simulink model "RTRCSystemValidation"  (R2022a)
settings: Solver=VariableStepAuto  StartTime=0.0  StopTime=TsimTime  FixedStep=Tsim  MaxStep=Tsim*100  RelTol=1e-5
undefined symbols (not defined in the file): Cdc, Fpwm, Jt, Kdw, Ke, Ki, Kii, Kiv, Kiw, Kp, Kpi, Kpv, Kpw, Krpm, Kt, Ktv, Ldc, Le, P, Rdc, Re, RPM_slope, Tload, Tpwm_buck, Vdc_c
libraries: simulink x10, slpidlib x1
settings Model: Creator=MasterGnome  LastModifiedBy=MasterGnome
settings SolverCC: ZeroCrossAlgorithm=Adaptive
settings DebuggingCC: IgnoredZcDiagnostic=none  UnconnectedInputMsg=warning  UnconnectedOutputMsg=warning  UnconnectedLineMsg=warning
settings RTWCC: DLArmComputeVersion=19.05

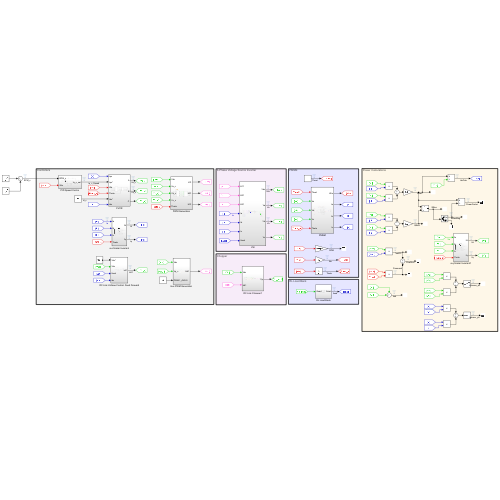
[thumbnail: Simulink's stored preview of the top-level diagram]
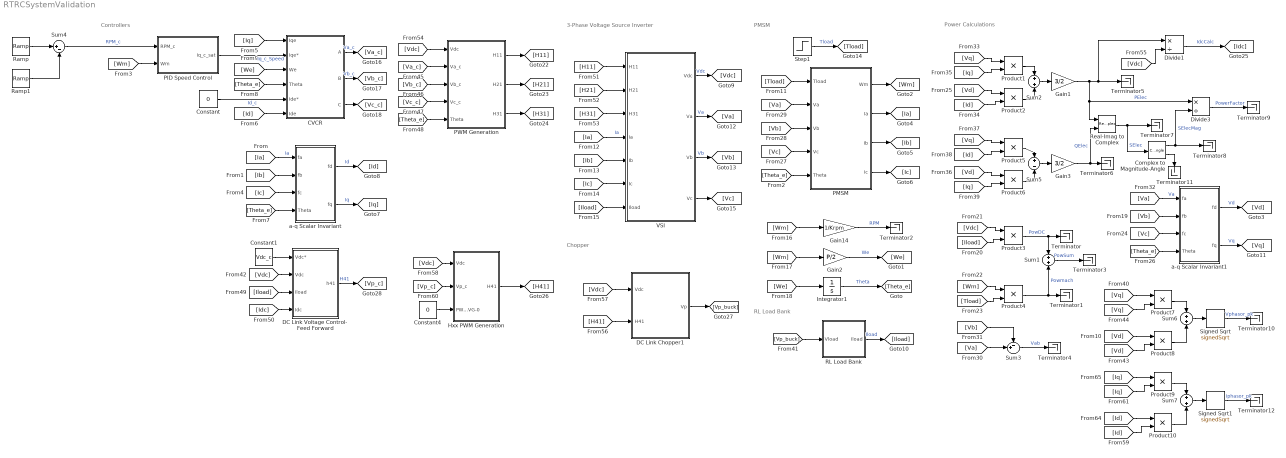
== system RTRCSystemValidation ==
  note: RL Load Bank
  note: Power Calculations
  note: PMSM
  note: Controllers
  note: 3-Phase Voltage Source Inverter
  note: Chopper
  CVCR : Subsystem
  Complex to Magnitude-Angle : ComplexToMagnitudeAngle
  Constant : Constant  Value=0
  Constant1 : Constant  Value=Vdc_c
  Constant4 : Constant  Value=0
  DC Link Chopper1 : Subsystem
  DC Link Voltage Control- Feed Forward : Subsystem
  Divide1 : Product  Inputs=*/
  Divide3 : Product  Inputs=*/
  Gain1 : Gain  Gain=3/2
  Gain14 : Gain  Gain=1/Krpm
  Gain2 : Gain  Gain=P/2
  Gain3 : Gain  Gain=3/2
  Hxx PWM Generation : Subsystem
  Integrator1 : Integrator
  PID Speed Control : Subsystem
  PMSM : Subsystem
  PWM Generation : Subsystem
  Product{1..10} (10 alike) : Product
  RL Load Bank : Subsystem
  Ramp : simulink/Sources/Ramp  slope=RPM_slope  start=RPM_Tstart  InitialOutput=0
  Ramp1 : simulink/Sources/Ramp  slope=RPM_slope  start=RPM_Tend  InitialOutput=0
  Real-Imag to Complex : RealImagToComplex
  Signed Sqrt : Sqrt  Operator=signedSqrt
  Signed Sqrt1 : Sqrt  Operator=signedSqrt
  Step1 : Step  Time=0.01  After=Tload  SampleTime=0
  Sum{1..2,6..7} (4 alike) : Sum  Inputs=+|+
  Sum3 : Sum  Inputs=-+|
  Sum4 : Sum  Inputs=|+-
  Sum5 : Sum  Inputs=+|-
  Terminator{,1..12} (13 alike) : Terminator
  VSI : Subsystem
  a-q Scalar Invariant : Subsystem
  a-q Scalar Invariant1 : Subsystem
  wires:
  Gain14/1 -> Terminator2/1  "RPM"
  PMSM/1(Wm) -> [Wm]
  Step1/1 -> [Tload]  "Tload"
  Gain2/1 -> [We]  "We"
  PMSM/2(Ia) -> [Ia]
  PMSM/3(Ib) -> [Ib]
  PMSM/4(Ic) -> [Ic]
  [Ia] -> a-q Scalar Invariant/1(fa)  "Ia"
  [Ib] -> a-q Scalar Invariant/2(fb)
  [Ic] -> a-q Scalar Invariant/3(fc)
  [Iq] -> CVCR/1(Iqe)
  [Id] -> CVCR/6(Ide)
  Integrator1/1 -> [Theta_e]  "Theta"
  [Theta_e] -> CVCR/4(Theta)
  [We] -> CVCR/3(We)
  Constant/1 -> CVCR/5(Ide*)  "Id_c"
  [Theta_e] -> PMSM/5(Theta)
  a-q Scalar Invariant/2(fq) -> [Iq]  "Iq"
  a-q Scalar Invariant/1(fd) -> [Id]  "Id"
  [Theta_e] -> a-q Scalar Invariant/4(Theta)
  Ramp/1 -> Sum4/1
  Ramp1/1 -> Sum4/2
  [Vdc] -> Product3/1
  [Iload] -> Product3/2
  Product3/1 -> Terminator/1, Sum1/1  "PowDC"
  Product4/1 -> Sum1/2, Terminator1/1  "Powmach"
  [Wm] -> Product4/1
  [Tload] -> Product4/2
  [Ib] -> VSI/5(Ib)
  [Ia] -> VSI/4(Ia)  "Ia"
  [Ic] -> VSI/6(Ic)
  VSI/1(Vdc) -> [Vdc]  "Vdc"
  [Tload] -> PMSM/1(Tload)
  Sum4/1 -> PID Speed Control/1(RPM_c)  "RPM_c"
  [Wm] -> PID Speed Control/2(Wm)
  PID Speed Control/1(Iq_c_sat) -> CVCR/2(Iqe*)  "Iq_c_Speed"
  [Wm] -> Gain14/1
  [Iload] -> VSI/7(Iload)
  [Wm] -> Gain2/1
  [We] -> Integrator1/1
  Sum1/1 -> Terminator3/1  "PowSum"
  Sum3/1 -> Terminator4/1  "Vab"
  [Vb] -> a-q Scalar Invariant1/2(fb)
  [Theta_e] -> a-q Scalar Invariant1/4(Theta)
  a-q Scalar Invariant1/1(fd) -> [Vd]  "Vd"
  [Vc] -> a-q Scalar Invariant1/3(fc)
  a-q Scalar Invariant1/2(fq) -> [Vq]  "Vq"
  [Va] -> a-q Scalar Invariant1/1(fa)  "Va"
  VSI/2(Va) -> [Va]  "Va"
  VSI/3(Vb) -> [Vb]  "Vb"
  VSI/4(Vc) -> [Vc]
  [Vc] -> PMSM/4(Vc)
  [Vb] -> PMSM/3(Vb)
  [Va] -> PMSM/2(Va)
  [Va] -> Sum3/2
  [Vb] -> Sum3/1
  [Iq] -> Product1/2
  [Vq] -> Product1/1
  [Id] -> Product2/2
  [Vd] -> Product2/1
  Product1/1 -> Sum2/1
  Product2/1 -> Sum2/2
  Sum2/1 -> Gain1/1
  Gain1/1 -> Divide1/1, Terminator5/1, Real-Imag to Complex/1, Divide3/1  "PElec"
  Product6/1 -> Sum5/2
  Product5/1 -> Sum5/1
  Gain3/1 -> Real-Imag to Complex/2, Terminator6/1  "QElec"
  [Vd] -> Product6/1
  [Vq] -> Product5/1
  Sum5/1 -> Gain3/1
  [Iq] -> Product6/2
  [Id] -> Product5/2
  Real-Imag to Complex/1 -> Complex to Magnitude-Angle/1, Terminator7/1  "SElec"
  Complex to Magnitude-Angle/1 -> Divide3/2, Terminator8/1  "SElecMag"
  Divide3/1 -> Terminator9/1  "PowerFactor"
  CVCR/3(C) -> [Vc_c]
  CVCR/2(B) -> [Vb_c]  "Vb_c"
  CVCR/1(A) -> [Va_c]  "Va_c"
  [H21] -> VSI/2(H21)
  [H31] -> VSI/3(H31)
  RL Load Bank/1(Iload) -> [Iload]  "Iload"
  [H11] -> VSI/1(H11)
  Complex to Magnitude-Angle/2 -> Terminator11/1
  [Vdc] -> PWM Generation/1(Vdc)
  [Va_c] -> PWM Generation/2(Va_c)
  [Vb_c] -> PWM Generation/3(Vb_c)
  [Vc_c] -> PWM Generation/4(Vc_c)
  [Theta_e] -> PWM Generation/5(Theta)
  PWM Generation/1(H11) -> [H11]
  PWM Generation/2(H21) -> [H21]
  PWM Generation/3(H31) -> [H31]
  [Vp_buck] -> RL Load Bank/1(Vload)
  Constant1/1 -> DC Link Voltage Control- Feed Forward/1(Vdc*)
  [Vdc] -> DC Link Voltage Control- Feed Forward/2(Vdc)
  [Iload] -> DC Link Voltage Control- Feed Forward/3(Iload)
  DC Link Voltage Control- Feed Forward/1(h41) -> [Vp_c]  "H41"
  [Vdc] -> Divide1/2
  [Idc] -> DC Link Voltage Control- Feed Forward/4(Idc)
  Divide1/1 -> [Idc]  "IdcCalc"
  Hxx PWM Generation/1(H41) -> [H41]
  Constant4/1 -> Hxx PWM Generation/3(PWM-1_AVG-0)
  [Vp_c] -> Hxx PWM Generation/2(Vp_c)
  [Vdc] -> Hxx PWM Generation/1(Vdc)
  [Vdc] -> DC Link Chopper1/1(Vdc)
  [H41] -> DC Link Chopper1/2(H41)
  DC Link Chopper1/1(Vp) -> [Vp_buck]
  [Vq] -> Product7/1
  [Vd] -> Product8/1
  Product7/1 -> Sum6/1
  Product8/1 -> Sum6/2
  [Vd] -> Product8/2
  [Vq] -> Product7/2
  Sum6/1 -> Signed Sqrt/1
  Signed Sqrt/1 -> Terminator10/1  "Vphasor_pk"
  Product9/1 -> Sum7/1
  Product10/1 -> Sum7/2
  Sum7/1 -> Signed Sqrt1/1
  Signed Sqrt1/1 -> Terminator12/1  "Iphasor_pk"
  [Iq] -> Product9/1
  [Id] -> Product10/1
  [Id] -> Product10/2
  [Iq] -> Product9/2

== system RTRCSystemValidation/CVCR ==
  Iqe : Inport
  Iqe* : Inport  Port=2
  We : Inport  Port=3
  Theta : Inport  Port=4
  Ide* : Inport  Port=5
  Ide : Inport  Port=6
  "CVCR " : Subsystem
  q-a Scalar Invariant : Subsystem
  A : Outport
  B : Outport  Port=2
  C : Outport  Port=3
  wires:
  q-a Scalar Invariant/3(c) -> C/1
  We/1 -> "CVCR "/3(We)
  Theta/1 -> q-a Scalar Invariant/3(theta)
  q-a Scalar Invariant/1(a) -> A/1
  q-a Scalar Invariant/2(b) -> B/1
  Iqe/1 -> "CVCR "/1(Iq)
  Iqe*/1 -> "CVCR "/2(Iq_c)
  Ide*/1 -> "CVCR "/4(Id_c)
  Ide/1 -> "CVCR "/5(Id)
  "CVCR "/1(Vqe) -> q-a Scalar Invariant/1(fq)  "Vq*"
  "CVCR "/2(Vde) -> q-a Scalar Invariant/2(fd)  "Vd*"

== system RTRCSystemValidation/DC Link Chopper1 ==
  Vdc : Inport
  H41 : Inport  Port=2
  Divide : Product  Inputs=**
  Vp : Outport
  wires:
  H41/1 -> [H41]
  [Vp] -> Vp/1
  Vdc/1 -> [Vdc]
  [H41] -> Divide/2
  [Vdc] -> Divide/1
  Divide/1 -> [Vp]  "Vp"

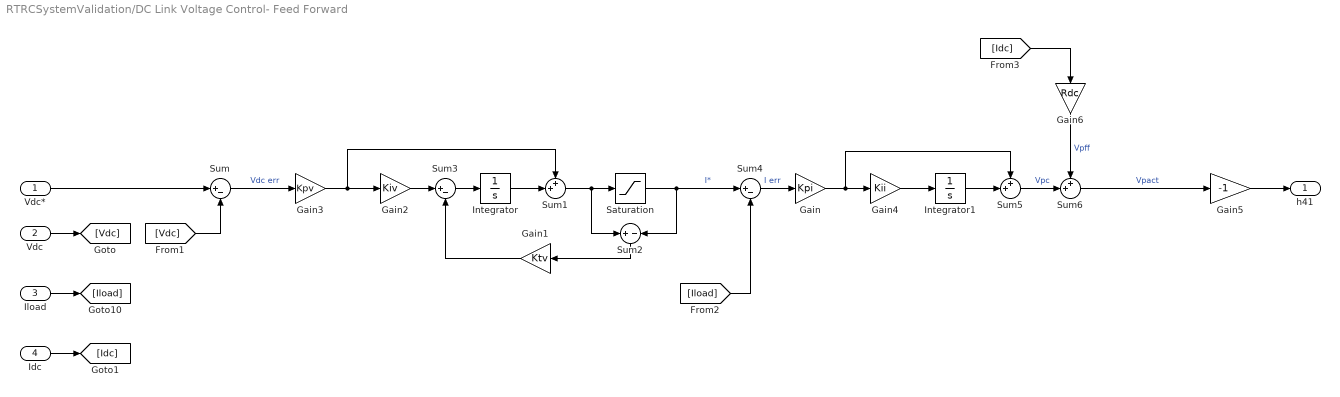
== system RTRCSystemValidation/DC Link Voltage Control- Feed Forward ==
  Vdc* : Inport
  Vdc : Inport  Port=2
  Iload : Inport  Port=3
  Idc : Inport  Port=4
  Gain : Gain  Gain=Kpi
  Gain1 : Gain  Gain=Ktv
  Gain2 : Gain  Gain=Kiv
  Gain3 : Gain  Gain=Kpv
  Gain4 : Gain  Gain=Kii
  Gain5 : Gain  Gain=-1
  Gain6 : Gain  Gain=Rdc
  Integrator : Integrator
  Integrator1 : Integrator
  Saturation : Saturate  UpperLimit=0  LowerLimit=-200
  Sum : Sum  Inputs=|+-
  Sum1 : Sum  Inputs=++|
  Sum2 : Sum  Inputs=+|-
  Sum3 : Sum  Inputs=|+-
  Sum4 : Sum  Inputs=|+-
  Sum5 : Sum  Inputs=++|
  Sum6 : Sum  Inputs=++|
  h41 : Outport
  wires:
  Sum/1 -> Gain3/1  "Vdc err"
  Gain3/1 -> Gain2/1, Sum1/1
  Sum1/1 -> Saturation/1, Sum2/1
  Gain2/1 -> Sum3/1
  Integrator/1 -> Sum1/2
  Sum3/1 -> Integrator/1
  Gain1/1 -> Sum3/2
  Sum2/1 -> Gain1/1
  Vdc*/1 -> Sum/1
  Sum4/1 -> Gain/1  "I err"
  Vdc/1 -> [Vdc]
  [Vdc] -> Sum/2
  Iload/1 -> [Iload]
  [Iload] -> Sum4/2
  Gain/1 -> Gain4/1, Sum5/1
  Gain4/1 -> Integrator1/1
  Integrator1/1 -> Sum5/2
  Gain5/1 -> h41/1
  Sum5/1 -> Sum6/2  "Vpc"
  Saturation/1 -> Sum4/1, Sum2/2  "I*"
  Idc/1 -> [Idc]
  Sum6/1 -> Gain5/1  "Vpact"
  [Idc] -> Gain6/1
  Gain6/1 -> Sum6/1  "Vpff"

== system RTRCSystemValidation/Hxx PWM Generation ==
  Vdc : Inport
  Vp_c : Inport  Port=2
  PWM-1_AVG-0 : Inport  Port=3
  Avg Model : Subsystem
  Switch7 : Switch  Criteria=u2 > Threshold  ZeroCross=off  SaturateOnIntegerOverflow=off  InputSameDT=off
  Switching Model : Subsystem
  H41 : Outport
  wires:
  [Vdc] -> Avg Model/1(Vdc)
  [Vp_c] -> Avg Model/2(Vp_c)
  Avg Model/1(H41_avg) -> [H41_avg]
  [Vdc] -> Switching Model/1(Vdc)
  [Vp_c] -> Switching Model/2(Vp_c)
  Switching Model/1(H41_pwm) -> [H41_pwm]
  [PWM_AVG] -> Switch7/2
  Switch7/1 -> [H41]
  [H41_pwm] -> Switch7/1
  [H41_avg] -> Switch7/3
  Vp_c/1 -> [Vp_c]
  Vdc/1 -> [Vdc]
  [H41] -> H41/1
  PWM-1_AVG-0/1 -> [PWM_AVG]

== system RTRCSystemValidation/PID Speed Control ==
  RPM_c : Inport
  Wm : Inport  Port=2
  Derivative : Derivative
  Gain1 : Gain  Gain=Kdw
  Gain10 : Gain  Gain=Kpw
  Gain11 : Gain  Gain=Krpm
  Gain2 : Gain  Gain=Kiw
  Integrator2 : Integrator
  Kt : Gain  Gain=100
  PID Controller : slpidlib/PID Controller  Controller=PID  Form=Parallel  TimeDomain=Continuous-time  UseExternalTs=off  SampleTime=-1  IntegratorMethod=Forward Euler  FilterMethod=Forward Euler  ControllerParametersSource=internal  P=Kpw  I=Kiw  UseKiTs=off  D=Kdw  N=100  UseFilter=on  TunerSelectOption=Transfer Function Based (PID Tuner App)  InitialConditionSource=internal  InitialConditionForIntegrator=0  InitialConditionForFilter=0  DifferentiatorICPrevScaledInput=0  ExternalReset=none  TrackingMode=off  Kt=1  LimitOutput=off  SatLimitsSource=internal  UpperSaturationLimit=inf  LowerSaturationLimit=-inf  LinearizeAsGain=on  AntiWindupMode=none  Kb=1  POutMin=[]  POutMax=[]  IOutMin=[]  IOutMax=[]  DOutMin=[]  DOutMax=[]  NOutMin=[]  NOutMax=[]  SumOutMin=[]  SumOutMax=[]  SaturationOutMin=[]  SaturationOutMax=[]  PParamMin=[]  PParamMax=[]  IParamMin=[]  IParamMax=[]  DParamMin=[]  DParamMax=[]  NParamMin=[]  NParamMax=[]  KbParamMin=[]  KbParamMax=[]  KtParamMin=[]  KtParamMax=[]  KbOutMin=[]  KbOutMax=[]  KtOutMin=[]  KtOutMax=[]  IntegratorOutMin=[]  IntegratorOutMax=[]  FilterOutMin=[]  FilterOutMax=[]  SumI1OutMin=[]  SumI1OutMax=[]  SumI2OutMin=[]  SumI2OutMax=[]  SumI3OutMin=[]  SumI3OutMax=[]  SumI4OutMin=[]  SumI4OutMax=[]  SumDOutMin=[]  SumDOutMax=[]  DifferentiatorOutMin=[]  DifferentiatorOutMax=[]  FilterDiffOutCoefMin=[]  FilterDiffOutCoefMax=[]  ReciprocalOutMin=[]  ReciprocalOutMax=[]  SumDenOutMin=[]  SumDenOutMax=[]  SumNumOutMin=[]  SumNumOutMax=[]  DivideOutMin=[]  DivideOutMax=[]  UdiffTsProdOutMin=[]  UdiffTsProdOutMax=[]  NTsProdOutMin=[]  NTsProdOutMax=[]  UintegralTsProdOutMin=[]  UintegralTsProdOutMax=[]  UngainTsProdOutMin=[]  UngainTsProdOutMax=[]  IntegratorContinuousStateAttributes=''  IntegratorStateMustResolveToSignalObject=off  IntegratorRTWStateStorageClass=Auto  FilterContinuousStateAttributes=''  FilterStateMustResolveToSignalObject=off  FilterRTWStateStorageClass=Auto  ParallelPVariant=InternalParameters  IdealPVariant=Disabled  IVariant=InternalParameters  DVariant=InternalParameters  IntegratorVariant=Continuous  SatVariant=Disabled  AWVariant=Passthrough  PCopyVariant=Disabled  TRVariant=Disabled  FdbkBlocksVariant=Forward  IdealPFdbkVariant=Disabled  SatFdbkVariant=Disabled  DerivativeFilterVariant=ContFilter  NVariant=InternalParameters  NCopyVariant=Disabled  FilterICVariant=InternalICsFilter  IntegratorICVariant=InternalICs  ExternalResetVariant=Disabled  TRSumVariant=Passthrough  SumFdbkVariant=Disabled  SumVariant=Sum_PID  TsampFilterVariant=InternalTs  TsampNgainVariant=Passthrough  TsampIntegralVariant=Passthrough  ExternalSaturationOutDataTypeStr=Inherit: Same as second input  aMode=0
  Saturation : Saturate  UpperLimit=150  LowerLimit=-150
  Saturation1 : Saturate  UpperLimit=150  LowerLimit=-150
  Sum1 : Sum  Inputs=+++
  Sum2 : Sum  Inputs=++|
  Sum3 : Sum  Inputs=|+-
  Sum4 : Sum  Inputs=+|-
  Sum5 : Sum  Inputs=|+-
  Sum9 : Sum  Inputs=|+-
  Iq_c_sat : Outport
  wires:
  Gain10/1 -> Sum1/1
  Wm/1 -> Sum9/2
  Gain1/1 -> Sum3/1
  Derivative/1 -> Sum1/2
  Gain11/1 -> Sum9/1
  RPM_c/1 -> Gain11/1
  Sum3/1 -> Derivative/1
  Sum5/1 -> Integrator2/1
  Saturation1/1 -> Sum1/3, Sum4/2
  Sum4/1 -> Kt/1
  Kt/1 -> Sum5/2
  Gain2/1 -> Sum5/1
  Integrator2/1 -> Sum2/2
  Sum9/1 -> PID Controller/1, Gain2/1, Gain1/1, Gain10/1
  Sum2/1 -> Sum4/1, Saturation1/1  "Iq_c"
  PID Controller/1 -> Saturation/1
  Saturation/1 -> Iq_c_sat/1  "Iq_c_sat"
  Sum1/1 -> ?  "Iq_c"

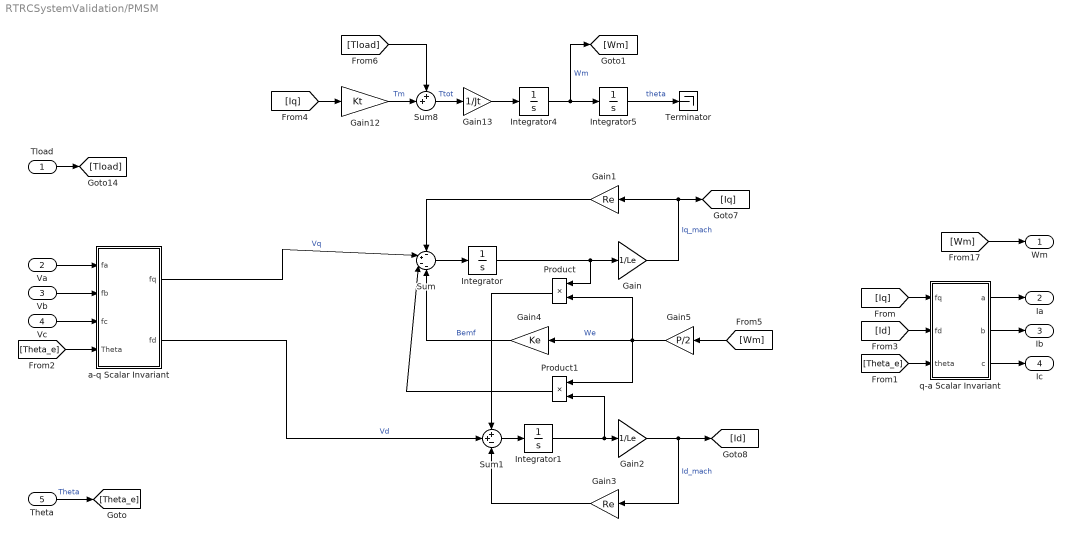
== system RTRCSystemValidation/PMSM ==
  Tload : Inport
  Va : Inport  Port=2
  Vb : Inport  Port=3
  Vc : Inport  Port=4
  Theta : Inport  Port=5
  Gain : Gain  Gain=1/Le
  Gain1 : Gain  Gain=Re
  Gain12 : Gain  Gain=Kt
  Gain13 : Gain  Gain=1/Jt
  Gain2 : Gain  Gain=1/Le
  Gain3 : Gain  Gain=Re
  Gain4 : Gain  Gain=Ke
  Gain5 : Gain  Gain=P/2
  Integrator{,1,4..5} (4 alike) : Integrator
  Product : Product
  Product1 : Product
  Sum : Sum  Inputs=-+--
  Sum1 : Sum  Inputs=++-
  Sum8 : Sum  Inputs=++|
  Terminator : Terminator
  a-q Scalar Invariant : Subsystem
  q-a Scalar Invariant : Subsystem
  Wm : Outport
  Ia : Outport  Port=2
  Ib : Outport  Port=3
  Ic : Outport  Port=4
  wires:
  Sum1/1 -> Integrator1/1
  Gain5/1 -> Product1/1, Product/2, Gain4/1  "We"
  Gain1/1 -> Sum/1
  Integrator4/1 -> [Wm], Integrator5/1  "Wm"
  Sum8/1 -> Gain13/1  "Ttot"
  Integrator1/1 -> Product1/2, Gain2/1
  Gain3/1 -> Sum1/3
  [Tload] -> Sum8/1
  Integrator/1 -> Product/1, Gain/1
  Gain13/1 -> Integrator4/1
  Gain4/1 -> Sum/4  "Bemf"
  Sum/1 -> Integrator/1
  Product/1 -> Sum1/1
  Integrator5/1 -> Terminator/1  "theta"
  Product1/1 -> Sum/3
  a-q Scalar Invariant/1(fq) -> Sum/2  "Vq"
  q-a Scalar Invariant/3(c) -> Ic/1
  q-a Scalar Invariant/1(a) -> Ia/1
  Gain2/1 -> [Id], Gain3/1  "Id_mach"
  q-a Scalar Invariant/2(b) -> Ib/1
  Gain/1 -> [Iq], Gain1/1  "Iq_mach"
  Vc/1 -> a-q Scalar Invariant/3(fc)
  Vb/1 -> a-q Scalar Invariant/2(fb)
  Va/1 -> a-q Scalar Invariant/1(fa)
  a-q Scalar Invariant/2(fd) -> Sum1/2  "Vd"
  [Theta_e] -> a-q Scalar Invariant/4(Theta)
  [Theta_e] -> q-a Scalar Invariant/3(theta)
  Theta/1 -> [Theta_e]  "Theta"
  [Iq] -> q-a Scalar Invariant/1(fq)
  [Id] -> q-a Scalar Invariant/2(fd)
  [Iq] -> Gain12/1
  Gain12/1 -> Sum8/2  "Tm"
  [Wm] -> Wm/1
  [Wm] -> Gain5/1
  Tload/1 -> [Tload]

== system RTRCSystemValidation/PWM Generation ==
  Vdc : Inport
  Va_c : Inport  Port=2
  Vb_c : Inport  Port=3
  Vc_c : Inport  Port=4
  Theta : Inport  Port=5
  "1-PWM, 0-AVG" : Constant  Value=0
  Hxx Avg PWM : Subsystem
  Modulation : Subsystem
  H11 : Outport
  H21 : Outport  Port=2
  H31 : Outport  Port=3
  wires:
  Modulation/1(Va_mod) -> [Va_mod]
  Modulation/2(Vb_mod) -> [Vb_mod]
  Hxx Avg PWM/1(H11) -> H11/1
  [Vb_mod] -> Hxx Avg PWM/3(Vb_mod)
  Hxx Avg PWM/2(H21) -> H21/1
  [Vc_mod] -> Hxx Avg PWM/4(Vc_mod)
  Modulation/3(Vc_mod) -> [Vc_mod]
  [Va_mod] -> Hxx Avg PWM/2(Va_mod)
  [Vdc] -> Hxx Avg PWM/1(Vdc)
  "1-PWM, 0-AVG"/1 -> Hxx Avg PWM/5(PWM-1_AVG-0)
  Hxx Avg PWM/3(H31) -> H31/1
  Vdc/1 -> [Vdc], Modulation/1(Vdc)
  Va_c/1 -> Modulation/2(Va_c)
  Vb_c/1 -> Modulation/3(Vb_c)
  Theta/1 -> Modulation/5(Theta)
  Vc_c/1 -> Modulation/4(Vc_c)

== system RTRCSystemValidation/RL Load Bank ==
  Vload : Inport
  Gain1 : Gain  Gain=-1
  Gain4 : Gain  Gain=1/Ldc
  Gain5 : Gain  Gain=Rdc
  Integrator2 : Integrator
  Sum6 : Sum  Inputs=|+-
  Iload : Outport
  wires:
  Gain5/1 -> Sum6/2
  Sum6/1 -> Gain4/1
  Vload/1 -> Sum6/1
  Gain4/1 -> Integrator2/1
  Integrator2/1 -> Gain1/1, Gain5/1  "Iload"
  Gain1/1 -> Iload/1

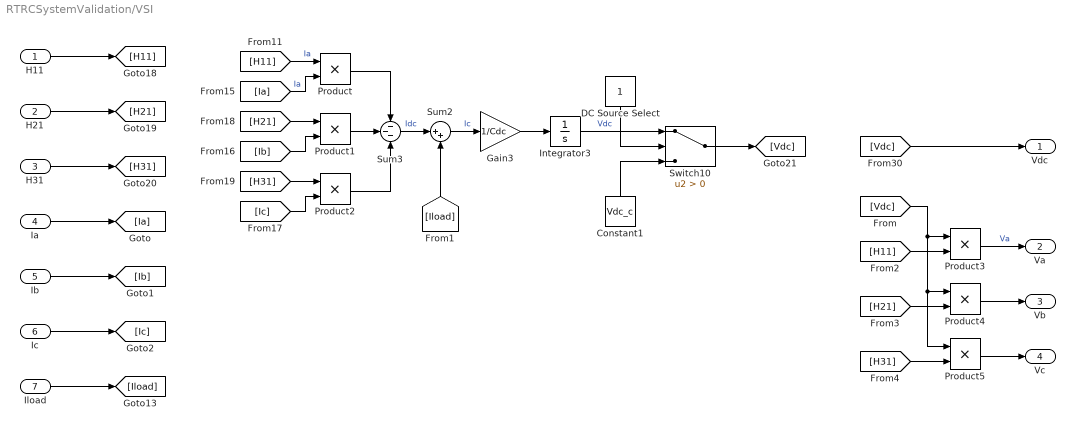
== system RTRCSystemValidation/VSI ==
  H11 : Inport
  H21 : Inport  Port=2
  H31 : Inport  Port=3
  Ia : Inport  Port=4
  Ib : Inport  Port=5
  Ic : Inport  Port=6
  Iload : Inport  Port=7
  Constant1 : Constant  Value=Vdc_c
  DC Source Select : Constant
  Gain3 : Gain  Gain=1/Cdc
  Integrator3 : Integrator  InitialCondition=Vdc_c/2
  Product{,1..5} (6 alike) : Product
  Sum2 : Sum  Inputs=|++
  Sum3 : Sum  Inputs=---
  Switch10 : Switch  Criteria=u2 > Threshold  ZeroCross=off  SaturateOnIntegerOverflow=off  InputSameDT=off
  Vdc : Outport
  Va : Outport  Port=2
  Vb : Outport  Port=3
  Vc : Outport  Port=4
  wires:
  Iload/1 -> [Iload]
  Sum3/1 -> Sum2/1  "Idc"
  H31/1 -> [H31]
  Sum2/1 -> Gain3/1  "Ic"
  H21/1 -> [H21]
  Product3/1 -> Va/1  "Va"
  [Ia] -> Product/2  "Ia"
  Product1/1 -> Sum3/2
  [Ib] -> Product1/2
  [H31] -> Product2/1
  [Ic] -> Product2/2
  Product2/1 -> Sum3/3
  [H21] -> Product1/1
  [Vdc] -> Vdc/1
  H11/1 -> [H11]
  [Vdc] -> Product3/1, Product5/1, Product4/1
  Product/1 -> Sum3/1
  [H11] -> Product/1  "Ia"
  Gain3/1 -> Integrator3/1
  Ib/1 -> [Ib]
  Ia/1 -> [Ia]
  Ic/1 -> [Ic]
  [Iload] -> Sum2/2
  Product4/1 -> Vb/1
  Product5/1 -> Vc/1
  Switch10/1 -> [Vdc]
  DC Source Select/1 -> Switch10/2
  Integrator3/1 -> Switch10/1  "Vdc"
  Constant1/1 -> Switch10/3
  [H11] -> Product3/2
  [H21] -> Product4/2
  [H31] -> Product5/2

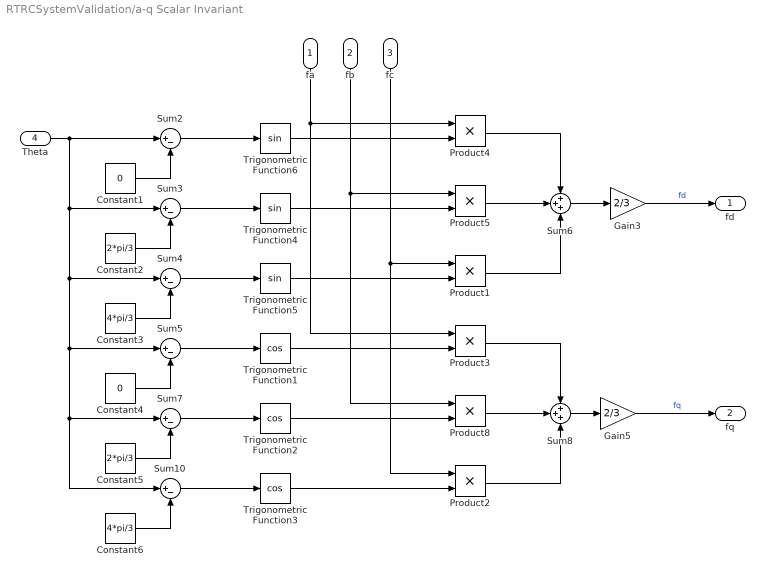
== system RTRCSystemValidation/a-q Scalar Invariant ==
  fa : Inport
  fb : Inport  Port=2
  fc : Inport  Port=3
  Theta : Inport  Port=4
  Constant1 : Constant  Value=0
  Constant2 : Constant  Value=2*pi/3
  Constant3 : Constant  Value=4*pi/3
  Constant4 : Constant  Value=0
  Constant5 : Constant  Value=2*pi/3
  Constant6 : Constant  Value=4*pi/3
  Gain3 : Gain  Gain=2/3
  Gain5 : Gain  Gain=2/3
  Product{1..5,8} (6 alike) : Product
  Sum{2..5,7,10} (6 alike) : Sum  Inputs=|+-
  Sum6 : Sum  Inputs=+++
  Sum8 : Sum  Inputs=+++
  Trigonometric Function1 : Trigonometry  Operator=cos
  Trigonometric Function2 : Trigonometry  Operator=cos
  Trigonometric Function3 : Trigonometry  Operator=cos
  Trigonometric Function4 : Trigonometry
  Trigonometric Function5 : Trigonometry
  Trigonometric Function6 : Trigonometry
  fd : Outport
  fq : Outport  Port=2
  wires:
  Product1/1 -> Sum6/3
  fc/1 -> Product2/1, Product1/1
  Sum4/1 -> Trigonometric Function5/1
  Constant5/1 -> Sum7/2
  Trigonometric Function4/1 -> Product5/2
  Sum7/1 -> Trigonometric Function2/1
  Constant6/1 -> Sum10/2
  Trigonometric Function3/1 -> Product2/2
  Theta/1 -> Sum10/1, Sum7/1, Sum5/1, Sum4/1, Sum3/1, Sum2/1
  Sum10/1 -> Trigonometric Function3/1
  Sum5/1 -> Trigonometric Function1/1
  Product2/1 -> Sum8/3
  Trigonometric Function2/1 -> Product8/2
  Product3/1 -> Sum8/1
  Constant3/1 -> Sum4/2
  Trigonometric Function6/1 -> Product4/2
  Product8/1 -> Sum8/2
  Trigonometric Function5/1 -> Product1/2
  Constant2/1 -> Sum3/2
  Sum3/1 -> Trigonometric Function4/1
  Sum8/1 -> Gain5/1
  Constant4/1 -> Sum5/2
  Constant1/1 -> Sum2/2
  Sum2/1 -> Trigonometric Function6/1
  fa/1 -> Product4/1, Product3/1
  Gain3/1 -> fd/1  "fd"
  Sum6/1 -> Gain3/1
  Trigonometric Function1/1 -> Product3/2
  Product4/1 -> Sum6/1
  Gain5/1 -> fq/1  "fq"
  fb/1 -> Product5/1, Product8/1
  Product5/1 -> Sum6/2

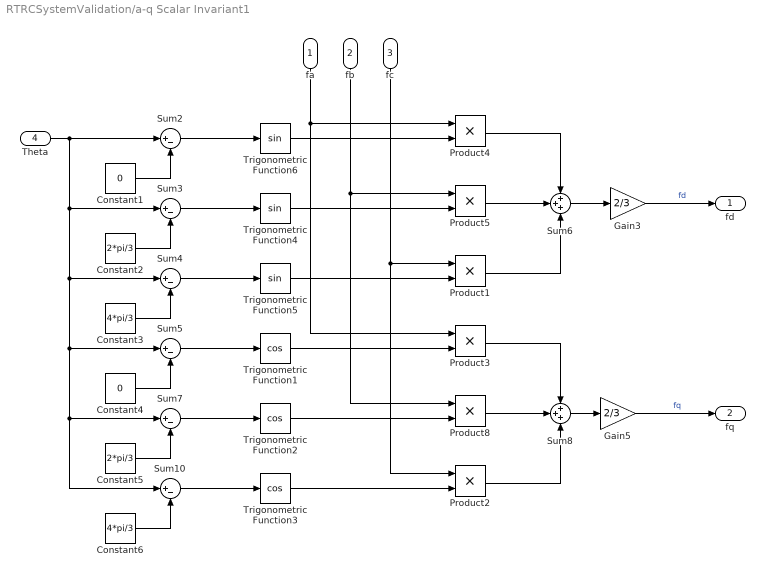
== system RTRCSystemValidation/a-q Scalar Invariant1 ==
  fa : Inport
  fb : Inport  Port=2
  fc : Inport  Port=3
  Theta : Inport  Port=4
  Constant1 : Constant  Value=0
  Constant2 : Constant  Value=2*pi/3
  Constant3 : Constant  Value=4*pi/3
  Constant4 : Constant  Value=0
  Constant5 : Constant  Value=2*pi/3
  Constant6 : Constant  Value=4*pi/3
  Gain3 : Gain  Gain=2/3
  Gain5 : Gain  Gain=2/3
  Product{1..5,8} (6 alike) : Product
  Sum{2..5,7,10} (6 alike) : Sum  Inputs=|+-
  Sum6 : Sum  Inputs=+++
  Sum8 : Sum  Inputs=+++
  Trigonometric Function1 : Trigonometry  Operator=cos
  Trigonometric Function2 : Trigonometry  Operator=cos
  Trigonometric Function3 : Trigonometry  Operator=cos
  Trigonometric Function4 : Trigonometry
  Trigonometric Function5 : Trigonometry
  Trigonometric Function6 : Trigonometry
  fd : Outport
  fq : Outport  Port=2
  wires:
  Product1/1 -> Sum6/3
  fc/1 -> Product2/1, Product1/1
  Sum4/1 -> Trigonometric Function5/1
  Constant5/1 -> Sum7/2
  Trigonometric Function4/1 -> Product5/2
  Sum7/1 -> Trigonometric Function2/1
  Constant6/1 -> Sum10/2
  Trigonometric Function3/1 -> Product2/2
  Theta/1 -> Sum10/1, Sum7/1, Sum5/1, Sum4/1, Sum3/1, Sum2/1
  Sum10/1 -> Trigonometric Function3/1
  Sum5/1 -> Trigonometric Function1/1
  Product2/1 -> Sum8/3
  Trigonometric Function2/1 -> Product8/2
  Product3/1 -> Sum8/1
  Constant3/1 -> Sum4/2
  Trigonometric Function6/1 -> Product4/2
  Product8/1 -> Sum8/2
  Trigonometric Function5/1 -> Product1/2
  Constant2/1 -> Sum3/2
  Sum3/1 -> Trigonometric Function4/1
  Sum8/1 -> Gain5/1
  Constant4/1 -> Sum5/2
  Constant1/1 -> Sum2/2
  Sum2/1 -> Trigonometric Function6/1
  fa/1 -> Product4/1, Product3/1
  Gain3/1 -> fd/1  "fd"
  Sum6/1 -> Gain3/1
  Trigonometric Function1/1 -> Product3/2
  Product4/1 -> Sum6/1
  Gain5/1 -> fq/1  "fq"
  fb/1 -> Product5/1, Product8/1
  Product5/1 -> Sum6/2

== system RTRCSystemValidation/CVCR/CVCR  ==
  Iq : Inport
  Iq_c : Inport  Port=2
  We : Inport  Port=3
  Id_c : Inport  Port=4
  Id : Inport  Port=5
  Gain6 : Gain  Gain=Ki
  Gain7 : Gain  Gain=Kp
  Gain8 : Gain  Gain=Ki
  Gain9 : Gain  Gain=Kp
  Integrator2 : Integrator
  Integrator3 : Integrator
  Product2 : Product
  Product3 : Product
  Sum2 : Sum  Inputs=++|
  Sum3 : Sum  Inputs=|++
  Sum4 : Sum  Inputs=-+|
  Sum5 : Sum  Inputs=|+-
  Sum6 : Sum  Inputs=|++
  Sum7 : Sum  Inputs=-+|
  Vqe : Outport
  Vde : Outport  Port=2
  wires:
  We/1 -> Product2/2, Product3/1
  Gain9/1 -> Product2/1, Gain8/1, Sum3/2
  Sum5/1 -> Gain9/1
  Integrator3/1 -> Sum3/1
  Product2/1 -> Sum6/2
  Gain7/1 -> Gain6/1, Sum2/1, Product3/2
  Product3/1 -> Sum7/1
  Sum6/1 -> Integrator2/1
  Id/1 -> Sum5/2
  Iq_c/1 -> Sum4/2
  Integrator2/1 -> Sum2/2
  Gain8/1 -> Sum7/2
  Sum4/1 -> Gain7/1
  Sum7/1 -> Integrator3/1
  Gain6/1 -> Sum6/1
  Iq/1 -> Sum4/1
  Sum2/1 -> Vqe/1  "Vqe"
  Id_c/1 -> Sum5/1
  Sum3/1 -> Vde/1  "Vde"

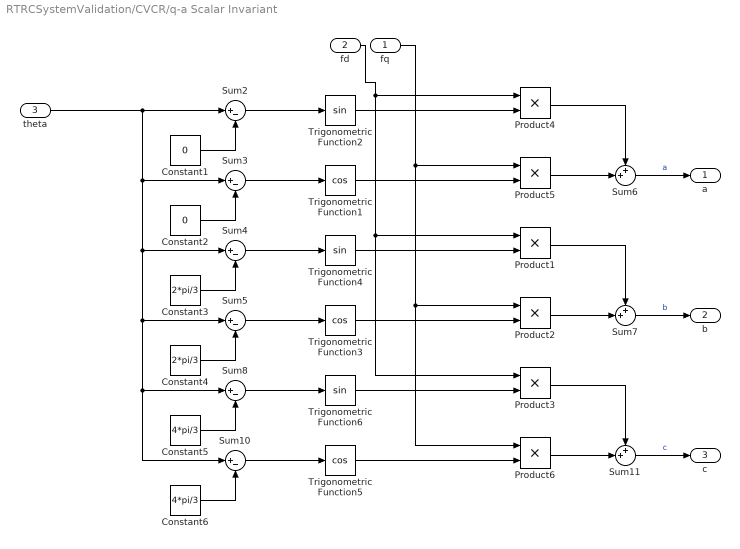
== system RTRCSystemValidation/CVCR/q-a Scalar Invariant ==
  fq : Inport
  fd : Inport  Port=2
  theta : Inport  Port=3
  Constant1 : Constant  Value=0
  Constant2 : Constant  Value=0
  Constant3 : Constant  Value=2*pi/3
  Constant4 : Constant  Value=2*pi/3
  Constant5 : Constant  Value=4*pi/3
  Constant6 : Constant  Value=4*pi/3
  Product{1..6} (6 alike) : Product
  Sum{2..5,8,10} (6 alike) : Sum  Inputs=|+-
  Sum11 : Sum  Inputs=++|
  Sum6 : Sum  Inputs=++|
  Sum7 : Sum  Inputs=++|
  Trigonometric Function1 : Trigonometry  Operator=cos
  Trigonometric Function2 : Trigonometry
  Trigonometric Function3 : Trigonometry  Operator=cos
  Trigonometric Function4 : Trigonometry
  Trigonometric Function5 : Trigonometry  Operator=cos
  Trigonometric Function6 : Trigonometry
  a : Outport
  b : Outport  Port=2
  c : Outport  Port=3
  wires:
  theta/1 -> Sum2/1, Sum3/1, Sum4/1, Sum5/1, Sum8/1, Sum10/1
  Trigonometric Function5/1 -> Product6/2
  Trigonometric Function6/1 -> Product3/2
  Constant4/1 -> Sum5/2
  Product1/1 -> Sum7/1
  Trigonometric Function2/1 -> Product4/2
  Product6/1 -> Sum11/2
  Sum10/1 -> Trigonometric Function5/1
  fd/1 -> Product3/1, Product1/1, Product4/1
  Sum3/1 -> Trigonometric Function1/1
  fq/1 -> Product6/1, Product2/1, Product5/1
  Product5/1 -> Sum6/2
  Trigonometric Function1/1 -> Product5/2
  Constant6/1 -> Sum10/2
  Sum8/1 -> Trigonometric Function6/1
  Sum2/1 -> Trigonometric Function2/1
  Sum4/1 -> Trigonometric Function4/1
  Constant1/1 -> Sum2/2
  Product2/1 -> Sum7/2
  Trigonometric Function4/1 -> Product1/2
  Sum5/1 -> Trigonometric Function3/1
  Trigonometric Function3/1 -> Product2/2
  Constant5/1 -> Sum8/2
  Sum6/1 -> a/1  "a"
  Constant3/1 -> Sum4/2
  Product3/1 -> Sum11/1
  Product4/1 -> Sum6/1
  Constant2/1 -> Sum3/2
  Sum11/1 -> c/1  "c"
  Sum7/1 -> b/1  "b"

== system RTRCSystemValidation/Hxx PWM Generation/Avg Model ==
  Vdc : Inport
  Vp_c : Inport  Port=2
  Constant2 : Constant  Commented=on  Value=2
  Constant6 : Constant  Value=0
  Constant7 : Constant
  Divide4 : Product  Inputs=/*
  Divide5 : Product  Commented=on  Inputs=/*
  Saturation Dynamic : simulink/Discontinuities/Saturation Dynamic  OutMin=[]  OutMax=[]  OutDataTypeStr=Inherit: Same as second input  OutDataType=fixdt(1, 16)  OutScaling=2^-10  DoSatur=off
  Sum5 : Sum  Inputs=++|
  H41_avg : Outport
  wires:
  Divide5/1 -> Sum5/1
  Constant7/1 -> Saturation Dynamic/1
  Constant2/1 -> Divide5/1
  Constant6/1 -> Saturation Dynamic/3
  Divide4/1 -> Saturation Dynamic/2
  Sum5/1 -> Divide4/2
  Vp_c/1 -> Sum5/2
  Vdc/1 -> Divide4/1, Divide5/2
  Saturation Dynamic/1 -> H41_avg/1

== system RTRCSystemValidation/Hxx PWM Generation/Switching Model ==
  Vdc : Inport
  Vp_c : Inport  Port=2
  Center Aligned : simulink/Sources/Repeating Sequence  rep_seq_t=[0 1/(2*Fpwm) 1/Fpwm]  rep_seq_y=[0 1 0]
  Constant3 : Constant  Commented=on  Value=2
  Delay : Delay  DelayLength=1  SampleTime=Tpwm_buck
  Divide1 : Product  Inputs=/*
  Divide2 : Product  Commented=on  Inputs=/*
  Edge Aligned : simulink/Sources/Repeating Sequence  Commented=on  rep_seq_t=[0 1/Fpwm]  rep_seq_y=[0 1]
  Relational Operator3 : RelationalOperator  Operator=>  OutDataTypeStr=boolean  ZeroCross=off  RndMeth=Simplest  InputSameDT=off
  Sum8 : Sum  Inputs=++|
  H41_pwm : Outport
  wires:
  Divide1/1 -> Relational Operator3/1  "Scaled"
  Center Aligned/1 -> Relational Operator3/2  "Carrier"
  Divide2/1 -> Sum8/1
  Vdc/1 -> Divide1/1, Divide2/2
  Edge Aligned/1 -> ?  "Carrier"
  Constant3/1 -> Divide2/1
  Sum8/1 -> Divide1/2
  Vp_c/1 -> Sum8/2
  Relational Operator3/1 -> Delay/1
  Delay/1 -> H41_pwm/1

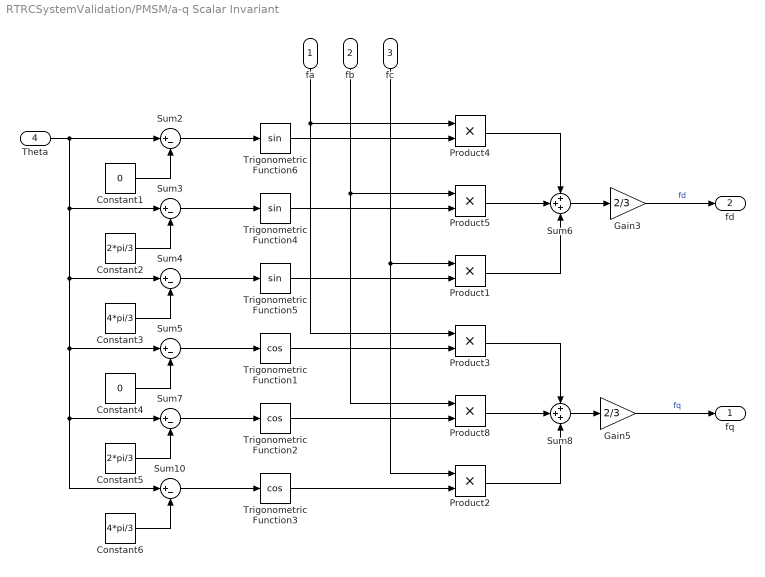
== system RTRCSystemValidation/PMSM/a-q Scalar Invariant ==
  fa : Inport
  fb : Inport  Port=2
  fc : Inport  Port=3
  Theta : Inport  Port=4
  Constant1 : Constant  Value=0
  Constant2 : Constant  Value=2*pi/3
  Constant3 : Constant  Value=4*pi/3
  Constant4 : Constant  Value=0
  Constant5 : Constant  Value=2*pi/3
  Constant6 : Constant  Value=4*pi/3
  Gain3 : Gain  Gain=2/3
  Gain5 : Gain  Gain=2/3
  Product{1..5,8} (6 alike) : Product
  Sum{2..5,7,10} (6 alike) : Sum  Inputs=|+-
  Sum6 : Sum  Inputs=+++
  Sum8 : Sum  Inputs=+++
  Trigonometric Function1 : Trigonometry  Operator=cos
  Trigonometric Function2 : Trigonometry  Operator=cos
  Trigonometric Function3 : Trigonometry  Operator=cos
  Trigonometric Function4 : Trigonometry
  Trigonometric Function5 : Trigonometry
  Trigonometric Function6 : Trigonometry
  fq : Outport
  fd : Outport  Port=2
  wires:
  Product1/1 -> Sum6/3
  fc/1 -> Product2/1, Product1/1
  Sum4/1 -> Trigonometric Function5/1
  Constant5/1 -> Sum7/2
  Trigonometric Function4/1 -> Product5/2
  Sum7/1 -> Trigonometric Function2/1
  Constant6/1 -> Sum10/2
  Trigonometric Function3/1 -> Product2/2
  Theta/1 -> Sum10/1, Sum7/1, Sum5/1, Sum4/1, Sum3/1, Sum2/1
  Sum10/1 -> Trigonometric Function3/1
  Sum5/1 -> Trigonometric Function1/1
  Product2/1 -> Sum8/3
  Trigonometric Function2/1 -> Product8/2
  Product3/1 -> Sum8/1
  Constant3/1 -> Sum4/2
  Trigonometric Function6/1 -> Product4/2
  Product8/1 -> Sum8/2
  Trigonometric Function5/1 -> Product1/2
  Constant2/1 -> Sum3/2
  Sum3/1 -> Trigonometric Function4/1
  Sum8/1 -> Gain5/1
  Constant4/1 -> Sum5/2
  Constant1/1 -> Sum2/2
  Sum2/1 -> Trigonometric Function6/1
  fa/1 -> Product4/1, Product3/1
  Gain3/1 -> fd/1  "fd"
  Sum6/1 -> Gain3/1
  Trigonometric Function1/1 -> Product3/2
  Product4/1 -> Sum6/1
  Gain5/1 -> fq/1  "fq"
  fb/1 -> Product5/1, Product8/1
  Product5/1 -> Sum6/2

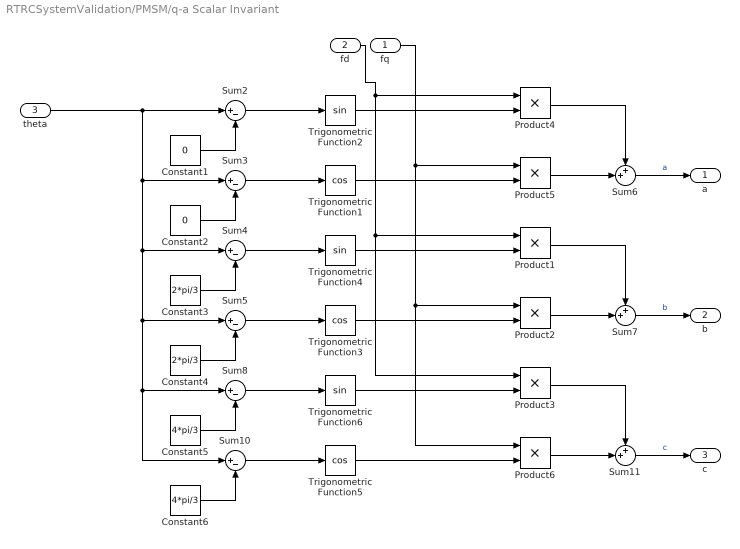
== system RTRCSystemValidation/PMSM/q-a Scalar Invariant ==
  fq : Inport
  fd : Inport  Port=2
  theta : Inport  Port=3
  Constant1 : Constant  Value=0
  Constant2 : Constant  Value=0
  Constant3 : Constant  Value=2*pi/3
  Constant4 : Constant  Value=2*pi/3
  Constant5 : Constant  Value=4*pi/3
  Constant6 : Constant  Value=4*pi/3
  Product{1..6} (6 alike) : Product
  Sum{2..5,8,10} (6 alike) : Sum  Inputs=|+-
  Sum11 : Sum  Inputs=++|
  Sum6 : Sum  Inputs=++|
  Sum7 : Sum  Inputs=++|
  Trigonometric Function1 : Trigonometry  Operator=cos
  Trigonometric Function2 : Trigonometry
  Trigonometric Function3 : Trigonometry  Operator=cos
  Trigonometric Function4 : Trigonometry
  Trigonometric Function5 : Trigonometry  Operator=cos
  Trigonometric Function6 : Trigonometry
  a : Outport
  b : Outport  Port=2
  c : Outport  Port=3
  wires:
  theta/1 -> Sum2/1, Sum3/1, Sum4/1, Sum5/1, Sum8/1, Sum10/1
  Trigonometric Function5/1 -> Product6/2
  Trigonometric Function6/1 -> Product3/2
  Constant4/1 -> Sum5/2
  Product1/1 -> Sum7/1
  Trigonometric Function2/1 -> Product4/2
  Product6/1 -> Sum11/2
  Sum10/1 -> Trigonometric Function5/1
  fd/1 -> Product3/1, Product1/1, Product4/1
  Sum3/1 -> Trigonometric Function1/1
  fq/1 -> Product6/1, Product2/1, Product5/1
  Product5/1 -> Sum6/2
  Trigonometric Function1/1 -> Product5/2
  Constant6/1 -> Sum10/2
  Sum8/1 -> Trigonometric Function6/1
  Sum2/1 -> Trigonometric Function2/1
  Sum4/1 -> Trigonometric Function4/1
  Constant1/1 -> Sum2/2
  Product2/1 -> Sum7/2
  Trigonometric Function4/1 -> Product1/2
  Sum5/1 -> Trigonometric Function3/1
  Trigonometric Function3/1 -> Product2/2
  Constant5/1 -> Sum8/2
  Sum6/1 -> a/1  "a"
  Constant3/1 -> Sum4/2
  Product3/1 -> Sum11/1
  Product4/1 -> Sum6/1
  Constant2/1 -> Sum3/2
  Sum11/1 -> c/1  "c"
  Sum7/1 -> b/1  "b"

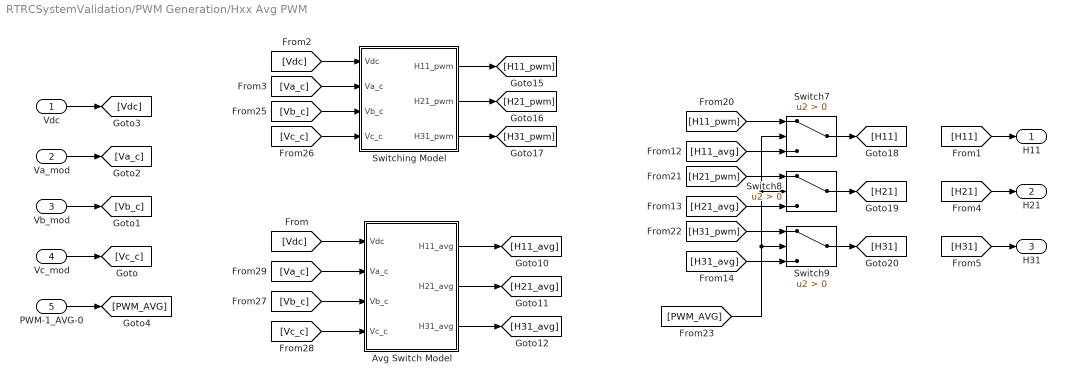
== system RTRCSystemValidation/PWM Generation/Hxx Avg PWM ==
  Vdc : Inport
  Va_mod : Inport  Port=2
  Vb_mod : Inport  Port=3
  Vc_mod : Inport  Port=4
  PWM-1_AVG-0 : Inport  Port=5
  Avg Switch Model : Subsystem
  Switch7 : Switch  Criteria=u2 > Threshold  ZeroCross=off  SaturateOnIntegerOverflow=off  InputSameDT=off
  Switch8 : Switch  Criteria=u2 > Threshold  ZeroCross=off  SaturateOnIntegerOverflow=off  InputSameDT=off
  Switch9 : Switch  Criteria=u2 > Threshold  ZeroCross=off  SaturateOnIntegerOverflow=off  InputSameDT=off
  Switching Model : Subsystem
  H11 : Outport
  H21 : Outport  Port=2
  H31 : Outport  Port=3
  wires:
  [Vdc] -> Avg Switch Model/1(Vdc)
  [Va_c] -> Avg Switch Model/2(Va_c)
  [Vb_c] -> Avg Switch Model/3(Vb_c)
  [Vc_c] -> Avg Switch Model/4(Vc_c)
  Avg Switch Model/1(H11_avg) -> [H11_avg]
  Avg Switch Model/2(H21_avg) -> [H21_avg]
  Avg Switch Model/3(H31_avg) -> [H31_avg]
  [Vdc] -> Switching Model/1(Vdc)
  [Va_c] -> Switching Model/2(Va_c)
  [Vb_c] -> Switching Model/3(Vb_c)
  [Vc_c] -> Switching Model/4(Vc_c)
  Switching Model/1(H11_pwm) -> [H11_pwm]
  Switching Model/2(H21_pwm) -> [H21_pwm]
  Switching Model/3(H31_pwm) -> [H31_pwm]
  [H31_pwm] -> Switch9/1
  [PWM_AVG] -> Switch9/2, Switch8/2, Switch7/2
  Switch8/1 -> [H21]
  Switch7/1 -> [H11]
  [H21_pwm] -> Switch8/1
  Switch9/1 -> [H31]
  [H21_avg] -> Switch8/3
  [H11_pwm] -> Switch7/1
  [H11_avg] -> Switch7/3
  [H31_avg] -> Switch9/3
  Vc_mod/1 -> [Vc_c]
  Va_mod/1 -> [Va_c]
  Vb_mod/1 -> [Vb_c]
  Vdc/1 -> [Vdc]
  [H21] -> H21/1
  [H31] -> H31/1
  [H11] -> H11/1
  PWM-1_AVG-0/1 -> [PWM_AVG]

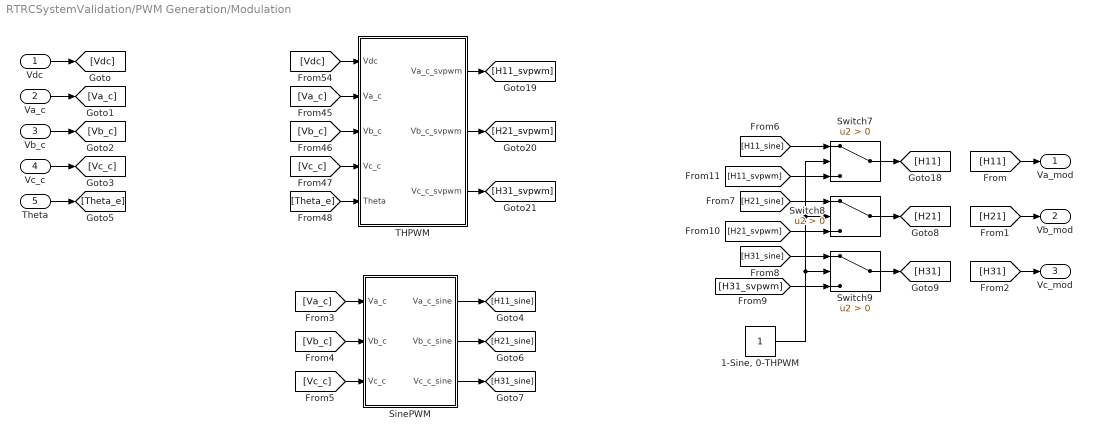
== system RTRCSystemValidation/PWM Generation/Modulation ==
  Vdc : Inport
  Va_c : Inport  Port=2
  Vb_c : Inport  Port=3
  Vc_c : Inport  Port=4
  Theta : Inport  Port=5
  "1-Sine, 0-THPWM" : Constant
  SinePWM : Subsystem
  Switch7 : Switch  Criteria=u2 > Threshold  ZeroCross=off  SaturateOnIntegerOverflow=off  InputSameDT=off
  Switch8 : Switch  Criteria=u2 > Threshold  ZeroCross=off  SaturateOnIntegerOverflow=off  InputSameDT=off
  Switch9 : Switch  Criteria=u2 > Threshold  ZeroCross=off  SaturateOnIntegerOverflow=off  InputSameDT=off
  THPWM : Subsystem
  Va_mod : Outport
  Vb_mod : Outport  Port=2
  Vc_mod : Outport  Port=3
  wires:
  Vdc/1 -> [Vdc]
  Va_c/1 -> [Va_c]
  Vb_c/1 -> [Vb_c]
  Vc_c/1 -> [Vc_c]
  Theta/1 -> [Theta_e]
  [Vdc] -> THPWM/1(Vdc)
  [Va_c] -> THPWM/2(Va_c)
  [Vb_c] -> THPWM/3(Vb_c)
  [Vc_c] -> THPWM/4(Vc_c)
  [Theta_e] -> THPWM/5(Theta)
  THPWM/1(Va_c_svpwm) -> [H11_svpwm]
  THPWM/2(Vb_c_svpwm) -> [H21_svpwm]
  THPWM/3(Vc_c_svpwm) -> [H31_svpwm]
  [H11] -> Va_mod/1
  [H21] -> Vb_mod/1
  [H31] -> Vc_mod/1
  [H21_sine] -> Switch8/1
  Switch9/1 -> [H31]
  [H11_svpwm] -> Switch7/3
  [H21_svpwm] -> Switch8/3
  [H11_sine] -> Switch7/1
  Switch7/1 -> [H11]
  [H31_svpwm] -> Switch9/3
  "1-Sine, 0-THPWM"/1 -> Switch9/2, Switch8/2, Switch7/2
  [H31_sine] -> Switch9/1
  Switch8/1 -> [H21]
  SinePWM/1(Va_c_sine) -> [H11_sine]
  SinePWM/2(Vb_c_sine) -> [H21_sine]
  SinePWM/3(Vc_c_sine) -> [H31_sine]
  [Vb_c] -> SinePWM/2(Vb_c)
  [Va_c] -> SinePWM/1(Va_c)
  [Vc_c] -> SinePWM/3(Vc_c)

== system RTRCSystemValidation/PWM Generation/Hxx Avg PWM/Avg Switch Model ==
  Vdc : Inport
  Va_c : Inport  Port=2
  Vb_c : Inport  Port=3
  Vc_c : Inport  Port=4
  Constant2 : Constant  Value=2
  Constant6 : Constant  Value=0
  Constant7 : Constant
  Divide{4..7} (4 alike) : Product  Inputs=/*
  Saturation Dynamic : simulink/Discontinuities/Saturation Dynamic  OutMin=[]  OutMax=[]  OutDataTypeStr=Inherit: Same as second input  OutDataType=fixdt(1, 16)  OutScaling=2^-10  DoSatur=off
  Saturation Dynamic1 : simulink/Discontinuities/Saturation Dynamic  OutMin=[]  OutMax=[]  OutDataTypeStr=Inherit: Same as second input  OutDataType=fixdt(1, 16)  OutScaling=2^-10  DoSatur=off
  Saturation Dynamic2 : simulink/Discontinuities/Saturation Dynamic  OutMin=[]  OutMax=[]  OutDataTypeStr=Inherit: Same as second input  OutDataType=fixdt(1, 16)  OutScaling=2^-10  DoSatur=off
  Sum1 : Sum  Inputs=++|
  Sum4 : Sum  Inputs=++|
  Sum5 : Sum  Inputs=++|
  H11_avg : Outport
  H21_avg : Outport  Port=2
  H31_avg : Outport  Port=3
  wires:
  Divide5/1 -> Sum1/1, Sum4/1, Sum5/1
  Constant7/1 -> Saturation Dynamic/1, Saturation Dynamic1/1, Saturation Dynamic2/1
  Constant2/1 -> Divide5/1
  Constant6/1 -> Saturation Dynamic2/3, Saturation Dynamic1/3, Saturation Dynamic/3
  Sum4/1 -> Divide6/2
  Divide4/1 -> Saturation Dynamic/2
  Divide6/1 -> Saturation Dynamic1/2
  Sum1/1 -> Divide7/2
  Saturation Dynamic2/1 -> H31_avg/1
  Divide7/1 -> Saturation Dynamic2/2
  Sum5/1 -> Divide4/2
  Va_c/1 -> Sum5/2
  Vdc/1 -> Divide7/1, Divide6/1, Divide4/1, Divide5/2
  Vc_c/1 -> Sum1/2
  Vb_c/1 -> Sum4/2
  Saturation Dynamic/1 -> H11_avg/1
  Saturation Dynamic1/1 -> H21_avg/1

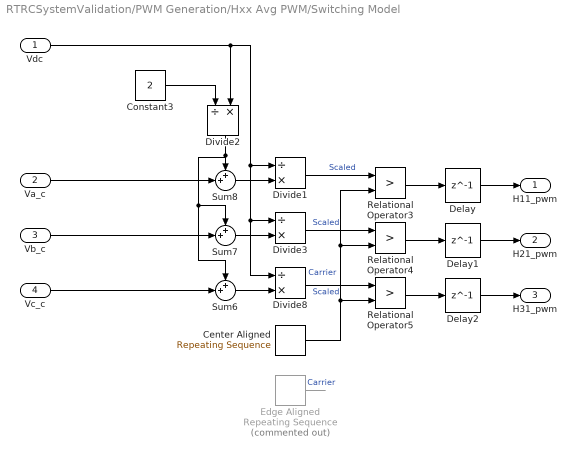
== system RTRCSystemValidation/PWM Generation/Hxx Avg PWM/Switching Model ==
  Vdc : Inport
  Va_c : Inport  Port=2
  Vb_c : Inport  Port=3
  Vc_c : Inport  Port=4
  Center Aligned : simulink/Sources/Repeating Sequence  rep_seq_t=[0 1/(2*Fpwm) 1/Fpwm]  rep_seq_y=[0 1 0]
  Constant3 : Constant  Value=2
  Delay : Delay  DelayLength=1
  Delay1 : Delay  DelayLength=1
  Delay2 : Delay  DelayLength=1
  Divide{1..3,8} (4 alike) : Product  Inputs=/*
  Edge Aligned : simulink/Sources/Repeating Sequence  Commented=on  rep_seq_t=[0 1/Fpwm]  rep_seq_y=[0 1]
  Relational Operator3 : RelationalOperator  Operator=>  OutDataTypeStr=boolean  ZeroCross=off  RndMeth=Simplest  InputSameDT=off
  Relational Operator4 : RelationalOperator  Operator=>  OutDataTypeStr=boolean  ZeroCross=off  RndMeth=Simplest  InputSameDT=off
  Relational Operator5 : RelationalOperator  Operator=>  OutDataTypeStr=boolean  ZeroCross=off  RndMeth=Simplest  InputSameDT=off
  Sum6 : Sum  Inputs=++|
  Sum7 : Sum  Inputs=++|
  Sum8 : Sum  Inputs=++|
  H11_pwm : Outport
  H21_pwm : Outport  Port=2
  H31_pwm : Outport  Port=3
  wires:
  Divide1/1 -> Relational Operator3/1  "Scaled"
  Center Aligned/1 -> Relational Operator3/2, Relational Operator4/2, Relational Operator5/2  "Carrier"
  Divide2/1 -> Sum6/1, Sum7/1, Sum8/1
  Vdc/1 -> Divide8/1, Divide3/1, Divide1/1, Divide2/2
  Relational Operator4/1 -> Delay1/1
  Edge Aligned/1 -> ?  "Carrier"
  Sum7/1 -> Divide3/2
  Constant3/1 -> Divide2/1
  Divide8/1 -> Relational Operator5/1  "Scaled"
  Sum6/1 -> Divide8/2
  Divide3/1 -> Relational Operator4/1  "Scaled"
  Sum8/1 -> Divide1/2
  Vc_c/1 -> Sum6/2
  Va_c/1 -> Sum8/2
  Vb_c/1 -> Sum7/2
  Relational Operator3/1 -> Delay/1
  Relational Operator5/1 -> Delay2/1
  Delay2/1 -> H31_pwm/1
  Delay/1 -> H11_pwm/1
  Delay1/1 -> H21_pwm/1

== system RTRCSystemValidation/PWM Generation/Modulation/SinePWM ==
  Va_c : Inport
  Vb_c : Inport  Port=2
  Vc_c : Inport  Port=3
  Va_c_sine : Outport
  Vb_c_sine : Outport  Port=2
  Vc_c_sine : Outport  Port=3
  wires:
  [Vc_c] -> [H31_sine]
  [Vb_c] -> [H21_sine]
  [Va_c] -> [H11_sine]
  Va_c/1 -> [Va_c]
  [H11_sine] -> Va_c_sine/1
  Vb_c/1 -> [Vb_c]
  Vc_c/1 -> [Vc_c]
  [H21_sine] -> Vb_c_sine/1
  [H31_sine] -> Vc_c_sine/1

== system RTRCSystemValidation/PWM Generation/Modulation/THPWM ==
  Vdc : Inport
  Va_c : Inport  Port=2
  Vb_c : Inport  Port=3
  Vc_c : Inport  Port=4
  Theta : Inport  Port=5
  Constant1 : Constant  Value=pi/6
  Constant3 : Constant  Value=9
  Divide : Product  Inputs=*/
  Divide1 : Product  Inputs=**
  Gain1 : Gain  Gain=3
  Sum{1..4} (4 alike) : Sum  Inputs=|+-
  Trigonometric Function6 : Trigonometry
  Va_c_svpwm : Outport
  Vb_c_svpwm : Outport  Port=2
  Vc_c_svpwm : Outport  Port=3
  wires:
  Vb_c/1 -> Sum1/1
  Sum1/1 -> Vb_c_svpwm/1
  Vc_c/1 -> Sum3/1
  Va_c/1 -> Sum2/1
  Sum3/1 -> Vc_c_svpwm/1
  Sum2/1 -> Va_c_svpwm/1
  Theta/1 -> Gain1/1
  Gain1/1 -> Sum4/1
  Vdc/1 -> Divide/1
  Constant3/1 -> Divide/2
  Divide/1 -> Divide1/1
  Trigonometric Function6/1 -> Divide1/2
  Divide1/1 -> Sum1/2, Sum2/2, Sum3/2  "zero_seq"
  Sum4/1 -> Trigonometric Function6/1
  Constant1/1 -> Sum4/2
